simulink model "aai"  (R2020a)
settings: Solver=FixedStepAuto  StartTime=0.0  StopTime=10.0  FixedStep=1e-3  RelTol=1e-3  EnableMultiTasking=on
undefined symbols (not defined in the file): D0, D10, D11, D12, D13, D2, D4, D5, D6, D7, D8, D9, PTA0, PTA2, PTB23, PTB9, PTC16, PTC2, PTC3, PTC4, PTD0, PTD1, PTD2, PTD3
libraries: frdmk64flib x12
settings Model: ExtModeTrigDuration=5  Creator=raymo  LastModifiedBy=raymo
settings OptimizationCC: EnhancedBackFolding=on  PassReuseOutputArgsAs=Individual arguments  ZeroExternalMemoryAtStartup=off  ZeroInternalMemoryAtStartup=off  MaxStackSize=64  OptimizeBlockOrder=speed  DifferentSizesBufferReuse=on  OptimizationCustomize=off  EfficientTunableParamExpr=on
settings DebuggingCC: ParameterTunabilityLossMsg=error
settings HardwareCC: ProdBitPerPointer=32  ProdBitPerSizeT=32  ProdBitPerPtrDiffT=32  ProdLargestAtomicInteger=Long  ProdLargestAtomicFloat=Double  ProdWordSize=32  ProdHWDeviceType=ARM Compatible->ARM Cortex
settings SFSimCC: MATLABDynamicMemAlloc=off
settings RTWCC: SystemTargetFile=ert.tlc  HardwareBoard=NXP FRDM-K64F  TemplateMakefile=ert_default_tmf  Toolchain=GNU Tools for ARM Embedded Processors
settings CodeAppCC: ForceParamTrailComments=on  IgnoreCustomStorageClasses=off  OperatorAnnotations=on  SimulinkDataObjDesc=on  SFDataObjDesc=on  InsertBlockDesc=on

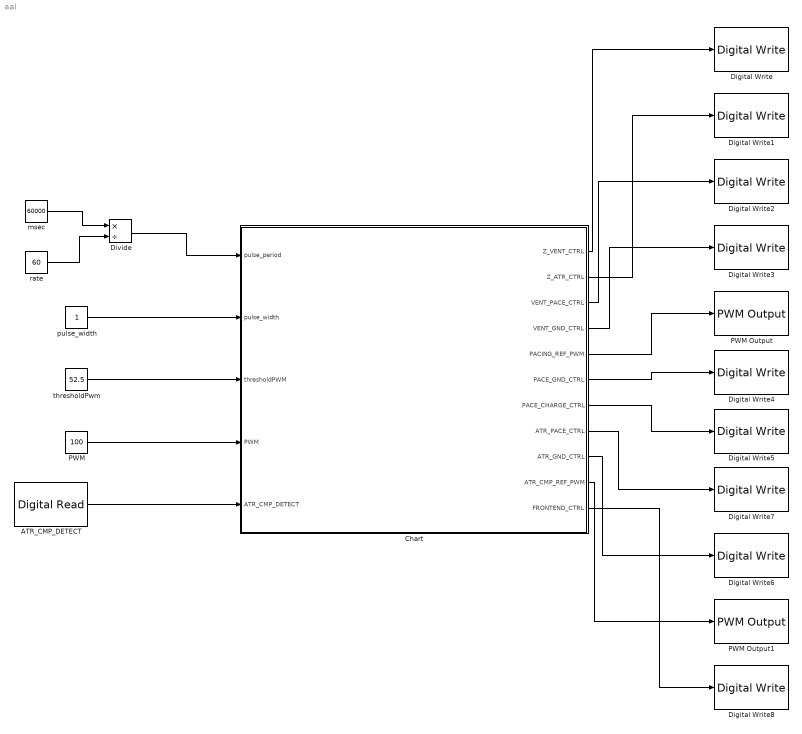
== system aai ==
  ATR_CMP_DETECT : frdmk64flib/Digital Read  Whichpin=PTC16 (D0)  SampleTime=-1
  Chart : Stateflow chart  TreatAsAtomicUnit=on
  Digital Write : frdmk64flib/Digital Write  Whichpin=PTC3 (D7)
  Digital Write1 : frdmk64flib/Digital Write  Whichpin=PTB23 (D4)
  Digital Write2 : frdmk64flib/Digital Write  Whichpin=PTC4 (D9)
  Digital Write3 : frdmk64flib/Digital Write  Whichpin=PTD3 (D12)
  Digital Write4 : frdmk64flib/Digital Write  Whichpin=PTD0 (D10)
  Digital Write5 : frdmk64flib/Digital Write  Whichpin=PTB9 (D2)
  Digital Write6 : frdmk64flib/Digital Write  Whichpin=PTD2 (D11)
  Digital Write7 : frdmk64flib/Digital Write  Whichpin=PTA0 (D8)
  Digital Write8 : frdmk64flib/Digital Write  Whichpin=PTD1 (D13)
  Divide : Product  Inputs=*/
  PWM : Constant  Value=100
  PWM Output : frdmk64flib/PWM Output  Whichpin=PTA2 (D5)  InitialFrequency=2000  InitialDutyCycle=50
  PWM Output1 : frdmk64flib/PWM Output  Whichpin=PTC2 (D6)  InitialFrequency=2000  InitialDutyCycle=50
  msec : Constant  Value=60000
  pulse_width : Constant
  rate : Constant  Value=60
  thresholdPwm : Constant  Value=52.5
  wires:
  ATR_CMP_DETECT/1 -> Chart/5(ATR_CMP_DETECT)
  thresholdPwm/1 -> Chart/3(thresholdPWM)
  Chart/5(PACING_REF_PWM) -> PWM Output/1
  Chart/10(ATR_CMP_REF_PWM) -> PWM Output1/1
  Chart/1(Z_VENT_CTRL) -> Digital Write/1
  Chart/2(Z_ATR_CTRL) -> Digital Write1/1
  Chart/3(VENT_PACE_CTRL) -> Digital Write2/1
  Chart/4(VENT_GND_CTRL) -> Digital Write3/1
  Chart/6(PACE_GND_CTRL) -> Digital Write4/1
  Chart/7(PACE_CHARGE_CTRL) -> Digital Write5/1
  Chart/9(ATR_GND_CTRL) -> Digital Write6/1
  Chart/8(ATR_PACE_CTRL) -> Digital Write7/1
  Chart/11(FRONTEND_CTRL) -> Digital Write8/1
  pulse_width/1 -> Chart/2(pulse_width)
  PWM/1 -> Chart/4(PWM)
  msec/1 -> Divide/1
  rate/1 -> Divide/2
  Divide/1 -> Chart/1(pulse_period)

== stateflow chart aai/Chart ==
  state Sense
    entry:
    %Set threshold
    ATR_CMP_REF_PWM = thresholdPWM;
    FRONTEND_CTRL = 1;
  state AVpacing
    entry:
    PACE_CHARGE_CTRL = 0;
    PACE_GND_CTRL = 1;
    ATR_PACE_CTRL = 1;
    ATR_GND_CTRL = 0;
    Z_ATR_CTRL = 0;
    Z_VENT_CTRL = 0;
    VENT_GND_CTRL = 0;
    VENT_PACE_CTRL = 0;
    PACING_REF_PWM = PWM;
    %Sensing
    FRONTEND_CTRL = 1;
  state ChargeDischarge
    entry:
    %C22
    ATR_PACE_CTRL = 0;
    VENT_PACE_CTRL = 0;
    PACING_REF_PWM = PWM;
    PACE_CHARGE_CTRL = 1;
    %C21
    PACE_GND_CTRL = 1;
    VENT_PACE_CTRL = 0;
    Z_ATR_CTRL = 0;
    Z_VENT_CTRL = 0;
    ATR_GND_CTRL = 1;
    VENT_GND_CTRL = 0;
    %Sensing
    FRONTEND_CTRL = 1;
  ChargeDischarge -> Sense : [after(pulse_period-pulse_width, msec)]
  (default) -> ChargeDischarge
  Sense -> (junction 11)
  (junction 11) -> ChargeDischarge [order 1] : [ATR_CMP_DETECT == 1]
  (junction 11) -> AVpacing [order 2] : [ATR_CMP_DETECT == 0]
  AVpacing -> ChargeDischarge : [after(pulse_width, msec)]
  data: pulse_period input; pulse_width input; thresholdPWM input; PWM input; Z_VENT_CTRL output; Z_ATR_CTRL output; VENT_PACE_CTRL output; VENT_GND_CTRL output; PACING_REF_PWM output; PACE_GND_CTRL output; PACE_CHARGE_CTRL output; ATR_PACE_CTRL output; ATR_GND_CTRL output; ATR_CMP_REF_PWM output; ATR_CMP_DETECT input; FRONTEND_CTRL output
